simulink model "CAN_Frequency_Effect_Anomalies"  (R2021a)
settings: Solver=FixedStepAuto  StartTime=0.0  StopTime=150  FixedStep=0.01  RelTol=1e-3
undefined symbols (not defined in the file or in its folder): canChannel
libraries: canlib x4, canmsglib x2
settings Model: Creator=saisa  LastModifiedBy=saisa

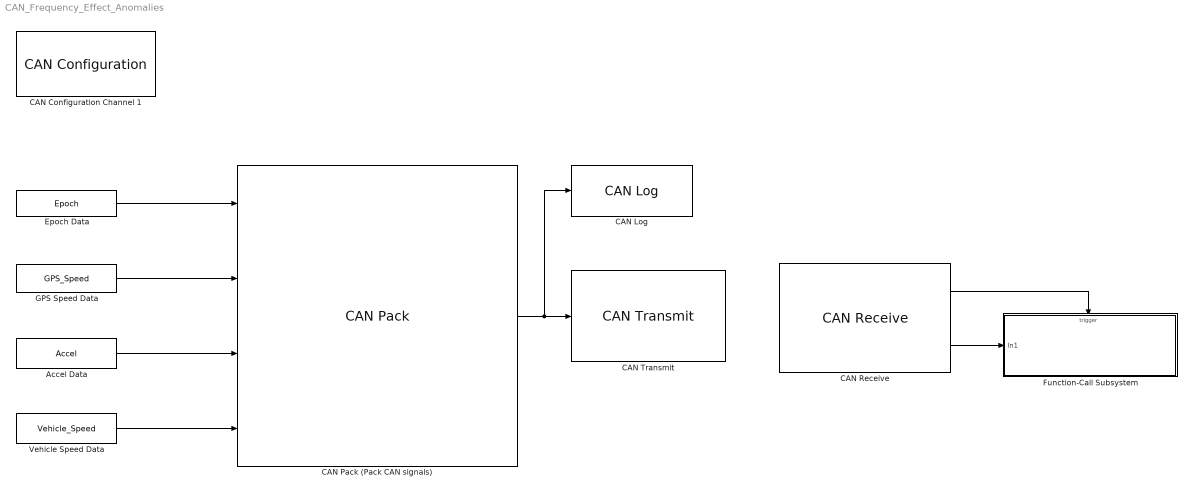
== system CAN_Frequency_Effect_Anomalies ==
  Accel Data : FromWorkspace  VariableName=Accel  OutDataTypeStr=double  SampleTime=0.01  Interpolate=off  ZeroCross=off  OutputAfterFinalValue=Holding final value
  CAN Configuration Channel 1 : canlib/CAN Configuration  BlockHandle=325.0006  Device=MathWorks Virtual 1 (Channel 1)  DeviceMenu=MathWorks Virtual 1 (Channel 1)  ObjConstructor=canChannel('MathWorks', 'Virtual 1', 1)  BusSpeed=500000  EnableBitParameters=off  AckMode=Normal
      settings: SourceProductBaseCode=VN
  CAN Log : canlib/CAN Log  BlockHandle=326.0006  FullPathFileName=Frequency_Effect.mat  FileName=Frequency_Effect.mat  VariableName=Frequency_Effect_Tx  MaxNumMessages=30000  LogFrom=Input port  DeviceMenu=Select a device  Device=Select a device  ObjConstructor=Select a constructor  SampleTime=0.01
      settings: SourceProductBaseCode=VN
  CAN Pack (Pack CAN signals) : canmsglib/CAN Pack  CANdbFile=C:\University\Course_Subjects\Semester_3\Study Project\Implementation\SPMD.dbc  MsgList=WheelSpeeds  MsgName=WheelSpeeds  MsgIDType=Standard (11-bit identifier)  MsgIdentifier=1200  MsgLength=8  Remote=off  ApplyMinMax=off  BusOutput=on  SignalInfo={'Epoch','0','16','LE','unsigned','Standard','0','0.01','0','0','30000';'GPS_Speed','16','16','LE','unsigned','Standard','0','0.01','-100','0','2000';'InVehicle_Longitudinal_Accel','48','16','LE','signed','Standard','0','0.01','-100','-2000','2000';'InVehicle_Longitudinal_Speed','32','16','LE','unsigned','Standard','0','0.01','-100','0','2000'}
      settings: SourceProductBaseCode=ME,XP,VN  DataFormat=CANdb specified signals
  CAN Receive : canlib/CAN Receive  BlockHandle=328.0006  Device=MathWorks Virtual 1 (Channel 1)  DeviceMenu=MathWorks Virtual 1 (Channel 1)  ObjConstructor=canChannel('MathWorks', 'Virtual 1', 1)  EnableStandardIDsFilter=off  StdIDsCombo=Allow all  StandardIDs=0  EnableExtendedIDsFilter=off  ExtIDsCombo=Allow all  ExtendedIDs=0  SampleTime=0.01  MsgsPerTimestep=all  InternalFilterUpdateStatus=on  BusOutput=on
      settings: SourceProductBaseCode=VN
  CAN Transmit : canlib/CAN Transmit  BlockHandle=329.0006  Device=MathWorks Virtual 1 (Channel 1)  DeviceMenu=MathWorks Virtual 1 (Channel 1)  ObjConstructor=canChannel('MathWorks', 'Virtual 1', 1)  EnableEventTransmit=off  EnablePeriodicTransmit=off  MessagePeriod=1.000
      settings: SourceProductBaseCode=VN
  Epoch Data : FromWorkspace  VariableName=Epoch  OutDataTypeStr=double  SampleTime=0.01  Interpolate=off  ZeroCross=off  OutputAfterFinalValue=Holding final value
  Function-Call Subsystem : Subsystem  TreatAsAtomicUnit=on
  GPS Speed Data : FromWorkspace  VariableName=GPS_Speed  OutDataTypeStr=double  SampleTime=0.01  Interpolate=off  ZeroCross=off  OutputAfterFinalValue=Holding final value
  Vehicle Speed Data : FromWorkspace  VariableName=Vehicle_Speed  OutDataTypeStr=double  SampleTime=0.01  Interpolate=off  ZeroCross=off  OutputAfterFinalValue=Holding final value
  wires:
  GPS Speed Data/1 -> CAN Pack (Pack CAN signals)/2
  Epoch Data/1 -> CAN Pack (Pack CAN signals)/1
  Vehicle Speed Data/1 -> CAN Pack (Pack CAN signals)/4
  Accel Data/1 -> CAN Pack (Pack CAN signals)/3
  CAN Receive/1 -> Function-Call Subsystem/Trigger
  CAN Receive/2 -> Function-Call Subsystem/1(In1)
  CAN Pack (Pack CAN signals)/1 -> CAN Log/1, CAN Transmit/1

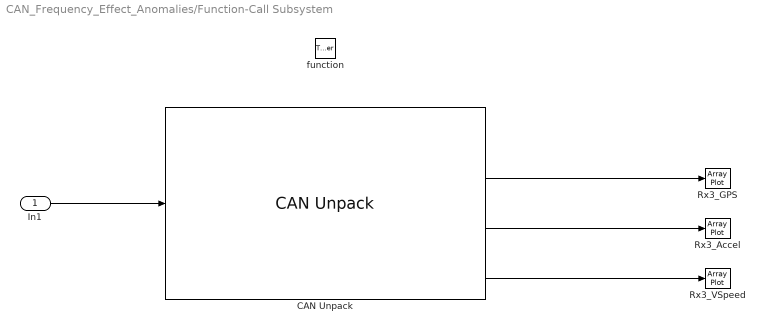
== system CAN_Frequency_Effect_Anomalies/Function-Call Subsystem ==
  In1 : Inport
  function : TriggerPort  TriggerType=function-call  VariantControl=(inherit)
  CAN Unpack : canmsglib/CAN Unpack  CANdbFile=C:\University\Course_Subjects\Semester_3\Study Project\Implementation\SPMD.dbc  MsgList=WheelSpeeds  MsgName=WheelSpeeds  MsgIDType=Standard (11-bit identifier)  MsgIdentifier=1200  MsgLength=8  SignalInfo={'Epoch','0','16','LE','unsigned','Standard','0','0.01','0','0','30000';'GPS_Speed','16','16','LE','unsigned','Standard','0','0.01','-100','0','2000';'InVehicle_Longitudinal_Accel','48','16','LE','signed','Standard','0','0.01','-100','-2000','2000';'InVehicle_Longitudinal_Speed','32','16','LE','unsigned','Standard','0','0.01','-100','0','2000'}  IDPort=off  TimestampPort=off  ErrorPort=off  RemotePort=off  LengthPort=off  StatusPort=off  ApplyMinMax=off
      settings: SourceProductBaseCode=ME,XP,VN  DataFormat=CANdb specified signals
  Rx3_Accel : ArrayPlot  WindowPosition=[240.000000,110.000000,800.000000,500.000000,]  DefaultConfigurationName=dsp.scopes.ArrayPlotBlockSpecification
  Rx3_GPS : ArrayPlot  WindowPosition=[240.000000,110.000000,800.000000,500.000000,]  DefaultConfigurationName=dsp.scopes.ArrayPlotBlockSpecification
  Rx3_VSpeed : ArrayPlot  WindowPosition=[240.000000,110.000000,800.000000,500.000000,]  DefaultConfigurationName=dsp.scopes.ArrayPlotBlockSpecification
  wires:
  In1/1 -> CAN Unpack/1
  CAN Unpack/2 -> Rx3_GPS/1
  CAN Unpack/3 -> Rx3_Accel/1
  CAN Unpack/4 -> Rx3_VSpeed/1
